simulink model "IMU_board_example_Sensors_grouped"  (R2015b)
settings: Solver=ode1  StartTime=0.0  StopTime=inf  FixedStep=.0005  RelTol=1e-3
undefined symbols (not defined in the file or in its folder): deg, s
libraries: qbmove_library_2015b x1, QB_pacer_lib x1, qbmove_library x1
settings Model: Creator=laurentio  LastModifiedBy=MattiaCP
settings DataIOCC: SaveFormat=Array
settings DebuggingCC: UnderspecifiedInitializationDetection=Classic  MergeDetectMultiDrivingBlocksExec=none  SolverPrmCheckMsg=warning  StateNameClashWarn=warning
settings HardwareCC: ProdBitPerPointer=32  ProdLargestAtomicFloat=None  ProdIntDivRoundTo=Undefined  ProdEndianess=Unspecified  ProdWordSize=32  ProdHWDeviceType=32-bit Generic
settings GRTTargetCC: GeneratePreprocessorConditionals=Disable all
settings ConfigComp: CovModelRefEnable=Off  CovSFcnEnable=off

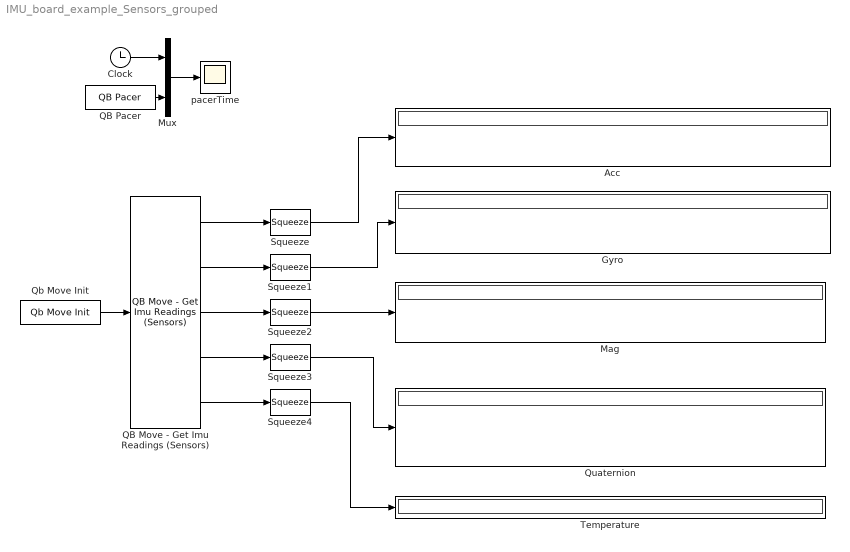
== system IMU_board_example_Sensors_grouped ==
  Acc : Display
  Clock : Clock
  Gyro : Display
  Mag : Display
  Mux : Mux  Inputs=2
  QB Move - Get Imu Readings (Sensors) : qbmove_library_2015b/QB Move - Get Imu Readings (Sensors)  ID=1  N_IMU=6  DAISY_CHAINING=off  ACC_UNITY=G  GYRO_UNITY=deg/s  MAG_UNITY=uT
  QB Pacer : QB_pacer_lib/QB Pacer  simTimePerRealTime=1
  Qb Move Init : qbmove_library/Qb Move Init  NUMBER_OF_COM='COM2'  BAUD_RATE_COM=2000000
  Quaternion : Display
  Squeeze{,1..4} (5 alike) : Squeeze
  Temperature : Display
  pacerTime : Scope
  wires:
  QB Pacer/1 -> Mux/2
  Clock/1 -> Mux/1
  Qb Move Init/1 -> QB Move - Get Imu Readings (Sensors)/1
  Mux/1 -> pacerTime/1
  QB Move - Get Imu Readings (Sensors)/1 -> Squeeze/1
  QB Move - Get Imu Readings (Sensors)/2 -> Squeeze1/1
  QB Move - Get Imu Readings (Sensors)/3 -> Squeeze2/1
  QB Move - Get Imu Readings (Sensors)/4 -> Squeeze3/1
  QB Move - Get Imu Readings (Sensors)/5 -> Squeeze4/1
  Squeeze/1 -> Acc/1
  Squeeze1/1 -> Gyro/1
  Squeeze2/1 -> Mag/1
  Squeeze3/1 -> Quaternion/1
  Squeeze4/1 -> Temperature/1
